simulink model "nh1"  (R2023b)
settings: Solver=ode113  StartTime=0.0  StopTime=10.0  RelTol=1e-10
values from neighbouring files (symbols this model uses):
  Ic = Iz + 2*Izz + 2*Mk*L^2    (= 6.63214583333)    [dane2nh.m]    (also in danenh.m)
  Ixx = 1/2*Mk*Rkola^2    (= 0.0140625)    [dane2nh.m]    (also in danenh.m)
  k1 = 10    [dane2nh.m]    (also in danenh.m)
  k2 = 15    [dane2nh.m]    (also in danenh.m)
  Kd = [100,0 ... (first row only)    [dane2nh.m]    (also in danenh.m = [1000,0; lab21.m = [D11,D12)
  L = 0.03    [dane2nh.m]    (also in danenh.m)
  Mc = Mp + 2*Mk    (= 106)    [dane2nh.m]    (also in danenh.m)
  Rkola = 0.075    [dane2nh.m]    (also in danenh.m)
  vd = 20    [dane2nh.m]    (also in danenh.m)
  wd = 4    [dane2nh.m]    (also in danenh.m)
settings Model: Creator=alozins2  LastModifiedBy=alozins2

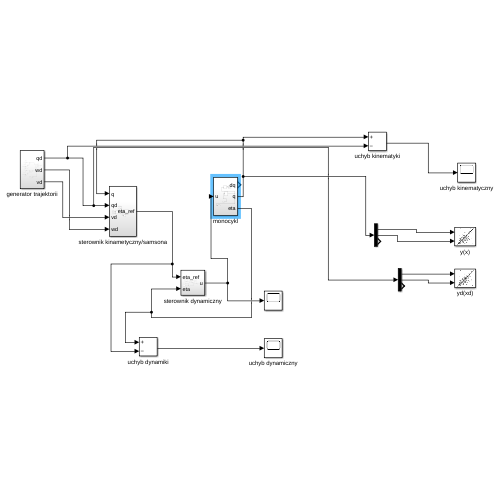
[thumbnail: Simulink's stored preview of the top-level diagram]
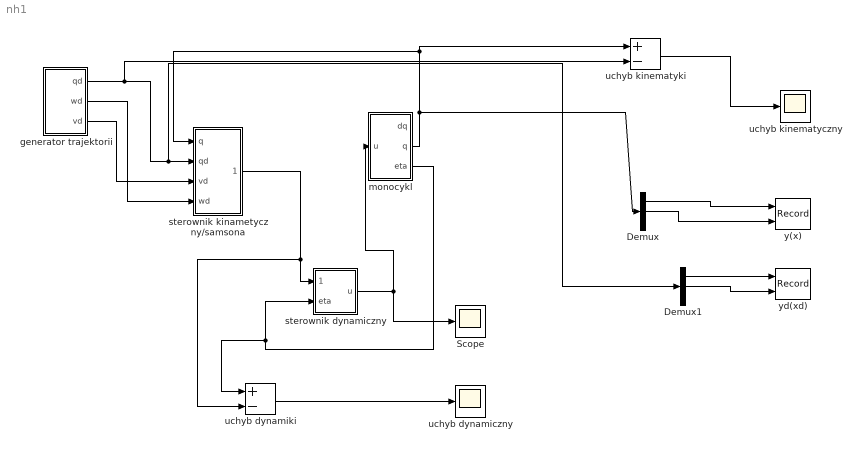
== system nh1 ==
  Demux : Demux  Outputs=3
  Demux1 : Demux  Outputs=3
  Scope : Scope
  generator trajektorii : Subsystem
  monocykl : Subsystem
  sterownik dynamiczny : Subsystem
  sterownik kinametyczny/samsona : Subsystem
  uchyb dynamiczny : Scope
  uchyb dynamiki : Sum  Inputs=+-
  uchyb kinematyczny : Scope
  uchyb kinematyki : Sum  Inputs=+-
  y(x) : Record  FileSettingsInternal="{\"entries\":[{\"content\":{\"excelSettings\":{\"content\":{},\"type\":\"Streamout.ExcelSettings\"}},\"type\":\"Streamout.FileSettingStorage\",\"uuid\":\"\"}],\"packageUris\":[\"http:\\/\\/schema.mathworks.com\\/mf0\\/streamout_blocks\\/R2020a\"],\"version\":\"1.0\"}"  Layout=[1 1]  SignalsInternal="{\"entries\":[{\"content\":{\"signals\":[{\"content\":{\"blockPath\":[],\"dimensions\":[1],\"domain\":\"\",\"lineColor\":\"#edb120\",\"plots\":[ 1 ],\"port\":1,\"signalID\":1,\"signalName\":\"Demux:1\"},\"type\":\"RecordBlkView.Signal\",\"uuid\":\"\"},{\"content\":{\"blockPath\":[],\"dimensions\":[1],\"domain\":\"\",\"lineColor\":\"#139fff\",\"plots\":[ 1 ],\"port\":2,\"signalID\":2,\"signalName\":\"Demux:2\"},\"type\":\"RecordBlkView.Signal\",\"uuid\":\"\"}]},\"type\":\"RecordBlkView.InputSignals\",\"uuid\":\"\"}],\"packageUris\":[\"http:\\/\\/schema.mathworks.com\\/mf0\\/streamout_blocks\\/R2020a\"],\"version\":\"1.0\"}"  VisualizationBindings="{\"xyplotplugin\":{\"info\":[{\"series\":[{\"bindingParametersList\":[{\"parameter\":\"X-Axis\",\"signalID\":1,\"signalName\":\"Demux:1\"},{\"parameter\":\"Y-Axis\",\"signalID\":2,\"signalName\":\"Demux:2\"}],\"seriesID\":0}],\"subplotID\":1}]}}"  CompatibilityTag=XY
  yd(xd) : Record  FileSettingsInternal="{\"entries\":[{\"content\":{\"excelSettings\":{\"content\":{},\"type\":\"Streamout.ExcelSettings\"}},\"type\":\"Streamout.FileSettingStorage\",\"uuid\":\"\"}],\"packageUris\":[\"http:\\/\\/schema.mathworks.com\\/mf0\\/streamout_blocks\\/R2020a\"],\"version\":\"1.0\"}"  Layout=[1 1]  SignalsInternal="{\"entries\":[{\"content\":{\"signals\":[{\"content\":{\"blockPath\":[],\"dimensions\":[1],\"domain\":\"\",\"lineColor\":\"#77ac30\",\"plots\":[ 1 ],\"port\":1,\"signalID\":1,\"signalName\":\"Demux1:1\"},\"type\":\"RecordBlkView.Signal\",\"uuid\":\"\"},{\"content\":{\"blockPath\":[],\"dimensions\":[1],\"domain\":\"\",\"lineColor\":\"#139fff\",\"plots\":[ 1 ],\"port\":2,\"signalID\":2,\"signalName\":\"Demux1:2\"},\"type\":\"RecordBlkView.Signal\",\"uuid\":\"\"}]},\"type\":\"RecordBlkView.InputSignals\",\"uuid\":\"\"}],\"packageUris\":[\"http:\\/\\/schema.mathworks.com\\/mf0\\/streamout_blocks\\/R2020a\"],\"version\":\"1.0\"}"  VisualizationBindings="{\"xyplotplugin\":{\"info\":[{\"series\":[{\"bindingParametersList\":[{\"parameter\":\"X-Axis\",\"signalID\":1,\"signalName\":\"Demux1:1\"},{\"parameter\":\"Y-Axis\",\"signalID\":2,\"signalName\":\"Demux1:2\"}],\"seriesID\":0}],\"subplotID\":1}]}}"  CompatibilityTag=XY
  wires:
  generator trajektorii/1(qd) -> uchyb kinematyki/2, Demux1/1, sterownik kinametyczny/samsona/2(qd)
  generator trajektorii/2(wd) -> sterownik kinametyczny/samsona/4(wd)
  generator trajektorii/3(vd) -> sterownik kinametyczny/samsona/3(vd)
  sterownik kinametyczny/samsona/1(eta_ref) -> sterownik dynamiczny/1(eta_ref), uchyb dynamiki/2
  sterownik dynamiczny/1(u) -> monocykl/1(u), Scope/1
  uchyb kinematyki/1 -> uchyb kinematyczny/1
  uchyb dynamiki/1 -> uchyb dynamiczny/1
  Demux/1 -> y(x)/1
  Demux/2 -> y(x)/2
  Demux1/1 -> yd(xd)/1
  Demux1/2 -> yd(xd)/2
  monocykl/3(eta) -> sterownik dynamiczny/2(eta), uchyb dynamiki/1
  monocykl/2(q) -> uchyb kinematyki/1, sterownik kinametyczny/samsona/1(q), Demux/1

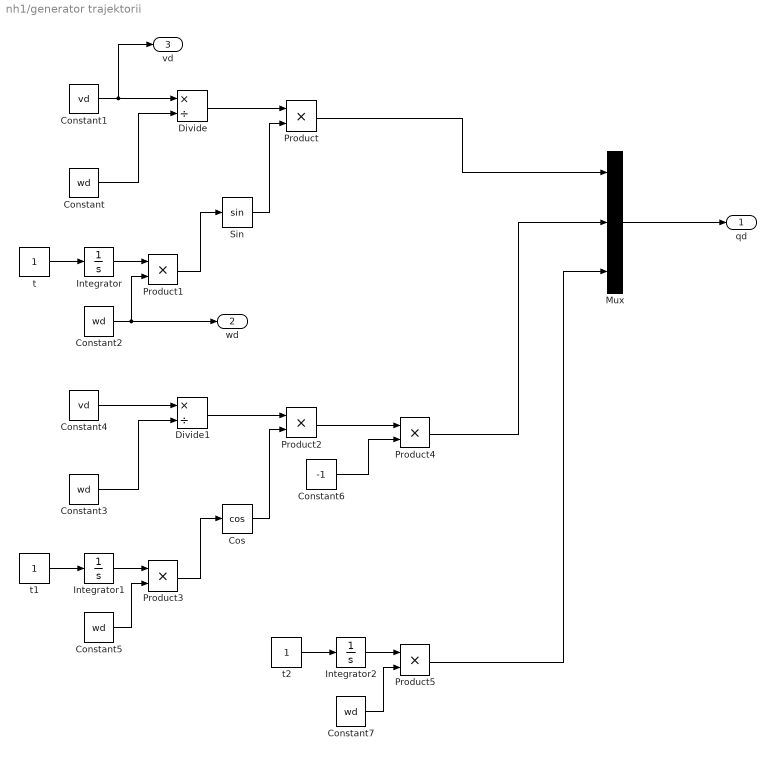
== system nh1/generator trajektorii ==
  Constant{,2..3,5,7} (5 alike) : Constant  Value=wd
  Constant1 : Constant  Value=vd
  Constant4 : Constant  Value=vd
  Constant6 : Constant  Value=-1
  Cos : Trigonometry  Operator=cos
  Divide : Product  Inputs=*/
  Divide1 : Product  Inputs=*/
  Integrator : Integrator
  Integrator1 : Integrator
  Integrator2 : Integrator
  Mux : Mux  Inputs=3
  Product{,1..5} (6 alike) : Product
  Sin : Trigonometry
  t : Constant
  t1 : Constant
  t2 : Constant
  qd : Outport
  wd : Outport  Port=2
  vd : Outport  Port=3
  wires:
  t1/1 -> Integrator1/1
  Product3/1 -> Cos/1
  Product5/1 -> Mux/3
  Integrator1/1 -> Product3/1
  Divide/1 -> Product/1
  Mux/1 -> qd/1
  Constant/1 -> Divide/2
  Product2/1 -> Product4/1
  Divide1/1 -> Product2/1
  Constant2/1 -> wd/1, Product1/2
  Constant3/1 -> Divide1/2
  Constant1/1 -> vd/1, Divide/1
  Cos/1 -> Product2/2
  Constant7/1 -> Product5/2
  Constant5/1 -> Product3/2
  Product4/1 -> Mux/2
  Product1/1 -> Sin/1
  Integrator2/1 -> Product5/1
  Constant6/1 -> Product4/2
  Product/1 -> Mux/1
  Constant4/1 -> Divide1/1
  t2/1 -> Integrator2/1
  Integrator/1 -> Product1/1
  Sin/1 -> Product/2
  t/1 -> Integrator/1

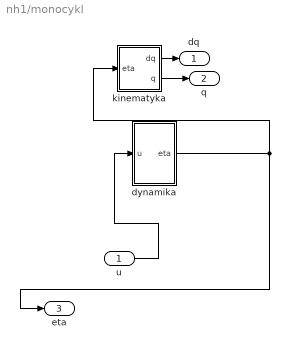
== system nh1/monocykl ==
  u : Inport
  dynamika : Subsystem
  kinematyka : Subsystem
  dq : Outport
  q : Outport  Port=2
  eta : Outport  Port=3
  wires:
  dynamika/1(eta) -> eta/1, kinematyka/1(eta)
  kinematyka/1(dq) -> dq/1
  kinematyka/2(q) -> q/1
  u/1 -> dynamika/1(u)

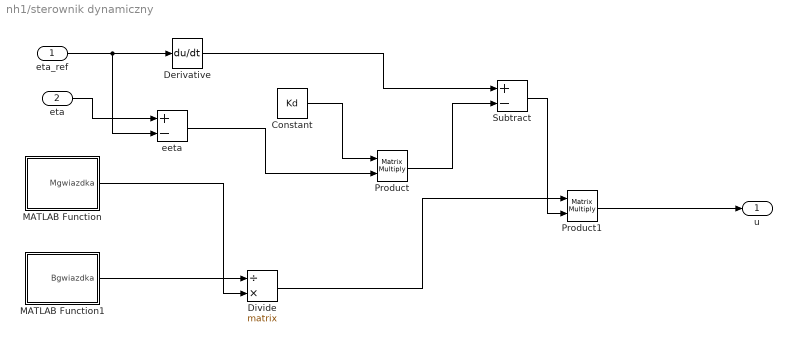
== system nh1/sterownik dynamiczny ==
  eta_ref : Inport
  eta : Inport  Port=2
  Constant : Constant  Value=Kd
  Derivative : Derivative
  Divide : Product  Inputs=/*  Multiplication=Matrix(*)
  MATLAB Function : MATLAB Function  TreatAsAtomicUnit=on
  MATLAB Function1 : MATLAB Function  TreatAsAtomicUnit=on
  Product : Product  Multiplication=Matrix(*)
  Product1 : Product  Multiplication=Matrix(*)
  Subtract : Sum  Inputs=+-
  eeta : Sum  Inputs=+-
  u : Outport
  wires:
  Product1/1 -> u/1
  Constant/1 -> Product/1
  Product/1 -> Subtract/2
  Derivative/1 -> Subtract/1
  MATLAB Function1/1(Bgwiazdka) -> Divide/1
  eta/1 -> eeta/1
  eeta/1 -> Product/2
  Divide/1 -> Product1/1
  MATLAB Function/1(Mgwiazdka) -> Divide/2
  Subtract/1 -> Product1/2
  eta_ref/1 -> eeta/2, Derivative/1

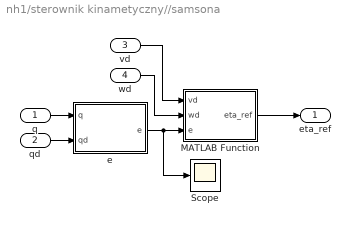
== system nh1/sterownik kinametyczny//samsona ==
  q : Inport
  qd : Inport  Port=2
  vd : Inport  Port=3
  wd : Inport  Port=4
  " e" : MATLAB Function  TreatAsAtomicUnit=on
  MATLAB Function : MATLAB Function  TreatAsAtomicUnit=on
  Scope : Scope
  eta_ref : Outport
  wires:
  q/1 -> " e"/1(q)
  " e"/1(e) -> Scope/1, MATLAB Function/3(e)
  qd/1 -> " e"/2(qd)
  vd/1 -> MATLAB Function/1(vd)
  wd/1 -> MATLAB Function/2(wd)
  MATLAB Function/1(eta_ref) -> eta_ref/1

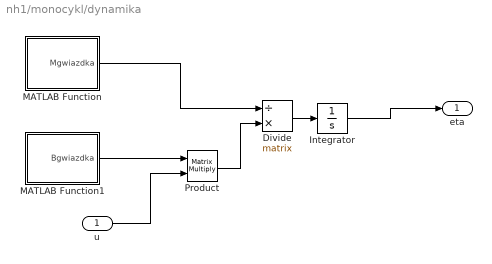
== system nh1/monocykl/dynamika ==
  u : Inport
  Divide : Product  Inputs=/*  Multiplication=Matrix(*)
  Integrator : Integrator  InitialCondition=[0;0]
  MATLAB Function : MATLAB Function  TreatAsAtomicUnit=on
  MATLAB Function1 : MATLAB Function  TreatAsAtomicUnit=on
  Product : Product  Multiplication=Matrix(*)
  eta : Outport
  wires:
  Integrator/1 -> eta/1
  MATLAB Function/1(Mgwiazdka) -> Divide/1
  Product/1 -> Divide/2
  u/1 -> Product/2
  Divide/1 -> Integrator/1
  MATLAB Function1/1(Bgwiazdka) -> Product/1

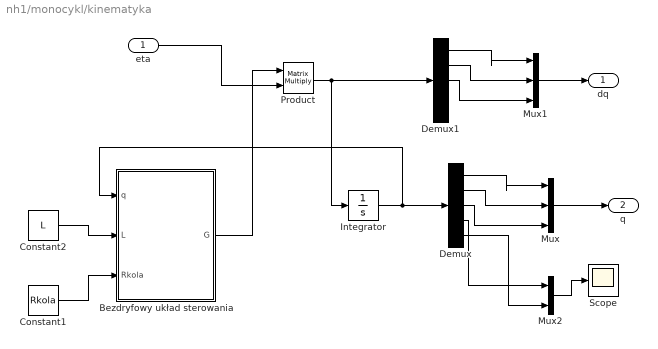
== system nh1/monocykl/kinematyka ==
  eta : Inport
  Bezdryfowy układ sterowania : MATLAB Function  TreatAsAtomicUnit=on
  Constant1 : Constant  Value=Rkola
  Constant2 : Constant  Value=L
  Demux : Demux  Outputs=5
  Demux1 : Demux  Outputs=5
  Integrator : Integrator  InitialCondition=[0;0;pi;0;0]
  Mux : Mux  Inputs=3
  Mux1 : Mux  Inputs=3
  Mux2 : Mux  Inputs=2
  Product : Product  Multiplication=Matrix(*)
  Scope : Scope
  dq : Outport
  q : Outport  Port=2
  wires:
  Integrator/1 -> Demux/1, Bezdryfowy układ sterowania/1(q)
  Product/1 -> Demux1/1, Integrator/1
  Constant1/1 -> Bezdryfowy układ sterowania/3(Rkola)
  Constant2/1 -> Bezdryfowy układ sterowania/2(L)
  eta/1 -> Product/2
  Bezdryfowy układ sterowania/1(G) -> Product/1
  Mux/1 -> q/1
  Demux/1 -> Mux/1
  Demux/2 -> Mux/2
  Demux/3 -> Mux/3
  Demux1/1 -> Mux1/1
  Demux1/3 -> Mux1/3
  Mux1/1 -> dq/1
  Demux1/2 -> Mux1/2
  Demux/4 -> Mux2/1
  Demux/5 -> Mux2/2
  Mux2/1 -> Scope/1

== matlab function nh1/sterownik kinametyczny//samsona/ e ==
  data: q input; e output; qd input
function e = fcn(q,qd)

x = q(1);
y = q(2);
teta = q(3);


xd = qd(1);
yd = qd(2);
tetad = qd(3);


e = [cos(teta)*(x-xd) + sin(teta)*(y-yd);
    -sin(teta)*(x-xd) + cos(teta)*(y-yd);
    teta-tetad];

== matlab function nh1/monocykl/kinematyka/Bezdryfowy układ sterowania ==
  data: q input; G output; L input; Rkola input
function G = bezdryfuklster(q,L,Rkola)
teta = q(3);

G = [cos(teta), 0;
    sin(teta),0;
    0,1;
    1/Rkola,L/Rkola;
    1/Rkola, -L/Rkola;];

== matlab function nh1/sterownik kinametyczny//samsona/MATLAB Function ==
  data: vd input; eta_ref output; wd input; e input; k1 parameter; k2 parameter
function eta_ref = fcn(vd,wd,e,k1, k2)

ex=e(1);
ey=e(2);
eteta=e(3);

v=vd*cos(eteta)-k1*ex;
if eteta<0.0001
    w = wd-vd*ey - k2*eteta;
else
    w= wd-vd*ey*(sin(eteta)/eteta)-k2*eteta;
end

eta_ref = [v;w];

== matlab function nh1/monocykl/dynamika/MATLAB Function ==
  data: Mc parameter; Ic parameter; Ixx parameter; Rkola parameter; L parameter; Mgwiazdka output
function Mgwiazdka = fcn(Mc, Ic, Ixx, Rkola, L)


Mgwiazdka = [Mc + (2*Ixx)/(Rkola^2), 0;
    0, Ic + (2*Ixx*L^2)/(Rkola^2)];

== matlab function nh1/monocykl/dynamika/MATLAB Function1 ==
  data: Bgwiazdka output; L parameter; Rkola parameter
function Bgwiazdka= fcn(L, Rkola)

Bgwiazdka=[1/Rkola,1/Rkola;
    L/Rkola, -L/Rkola];

== matlab function nh1/sterownik dynamiczny/MATLAB Function ==
  data: Mc parameter; Ic parameter; Ixx parameter; Rkola parameter; L parameter; Mgwiazdka output
function Mgwiazdka = fcn(Mc, Ic, Ixx, Rkola, L)


Mgwiazdka = [Mc + (2*Ixx)/(Rkola^2), 0;
    0, Ic + (2*Ixx*L^2)/(Rkola^2)];

== matlab function nh1/sterownik dynamiczny/MATLAB Function1 ==
  data: Bgwiazdka output; L parameter; Rkola parameter
function Bgwiazdka= fcn(L, Rkola)

Bgwiazdka=[1/Rkola,1/Rkola;
    L/Rkola, -L/Rkola];
